simulink model "Pitch_rate_command"  (R2025b)
settings: Solver=VariableStepAuto  StartTime=0.0  StopTime=10.0  RelTol=1e-3
settings Model: Creator=Jakub  LastModifiedBy=Jakub

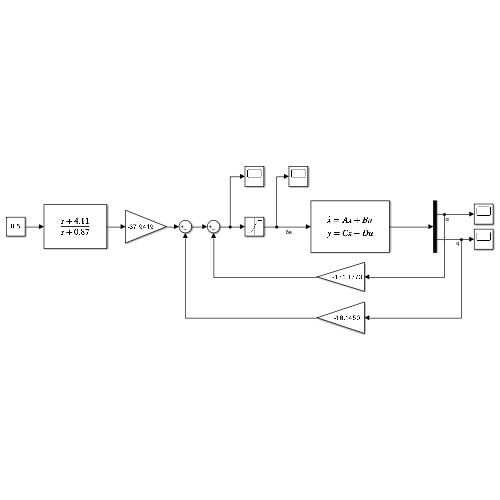
[thumbnail: Simulink's stored preview of the top-level diagram]
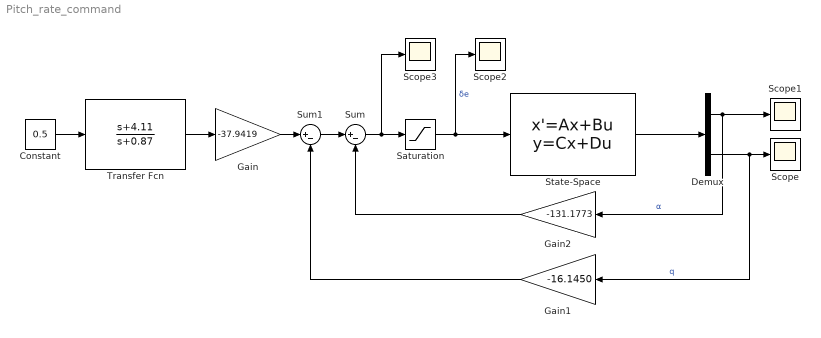
== system Pitch_rate_command ==
  Constant : Constant  Value=0.5
  Demux : Demux  Outputs=2
  Gain : Gain  Gain=-37.9419
  Gain1 : Gain  Gain=-16.1450
  Gain2 : Gain  Gain=-131.1773
  Saturation : Saturate  UpperLimit=25  LowerLimit=-25
  Scope{,1..3} (4 alike) : Scope
      Scope settings: ActiveDisplayYMinimum=-1.0151861408242542  ActiveDisplayYMaximum=2.9992471600607318
      Scope1 settings: ActiveDisplayYMinimum=-16.109168396732962  ActiveDisplayYMaximum=13.220070382193176
      Scope2 settings: ActiveDisplayYMinimum=-38.642737383135383  ActiveDisplayYMaximum=-4.4359502208090875  DataLoggingVariableName=ScopeData2
      Scope3 settings: ActiveDisplayYMinimum=-53.980593403455977  ActiveDisplayYMaximum=31.627525766338984  DataLoggingVariableName=ScopeData3
  State-Space : StateSpace  A=[-0.9006 0.9299; -2.6378 -1.2238]  B=[-0.0019; -0.1928]  C=[1 0; 0 1]  D=[0; 0]  InitialCondition=[0; 0]
  Sum : Sum  Inputs=|+-
  Sum1 : Sum  Inputs=|+-
  Transfer Fcn : TransferFcn  Numerator=[1 4.11]  Denominator=[1 0.87]
  wires:
  Constant/1 -> Transfer Fcn/1
  Transfer Fcn/1 -> Gain/1
  Saturation/1 -> Scope2/1, State-Space/1  "δe"
  Gain/1 -> Sum1/1
  State-Space/1 -> Demux/1
  Gain1/1 -> Sum1/2
  Sum/1 -> Scope3/1, Saturation/1
  Sum1/1 -> Sum/1
  Demux/1 -> Gain2/1, Scope1/1  "α"
  Demux/2 -> Gain1/1, Scope/1  "q"
  Gain2/1 -> Sum/2
